simulink model "quaternion_pid_development_sim"  (R2025b)
settings: Solver=FixedStepAuto  StartTime=0.0  StopTime=tspan  FixedStep=dt_sim  RelTol=1e-3
values from neighbouring files (symbols this model uses):
  dt_data = round((dt_data_target/dt_sim))*dt_sim    [quaternion_pid_development.m]
  Kd = 0    [quaternion_pid_development.m]
  Ki = 0    [quaternion_pid_development.m]
  Kp = 3    [quaternion_pid_development.m]
  qib_0 = eulToQuat(Eul_0)    [quaternion_pid_development.m]
  qib_u = squeeze(results.qib_u.Data)'    [quaternion_pid_development.m]
settings Model: Creator=koryh  LastModifiedBy=koryh

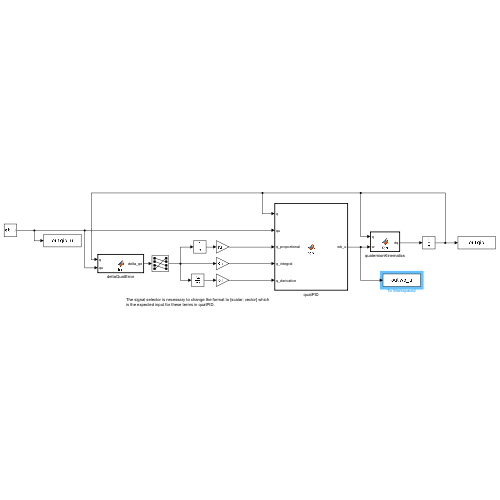
[thumbnail: Simulink's stored preview of the top-level diagram]
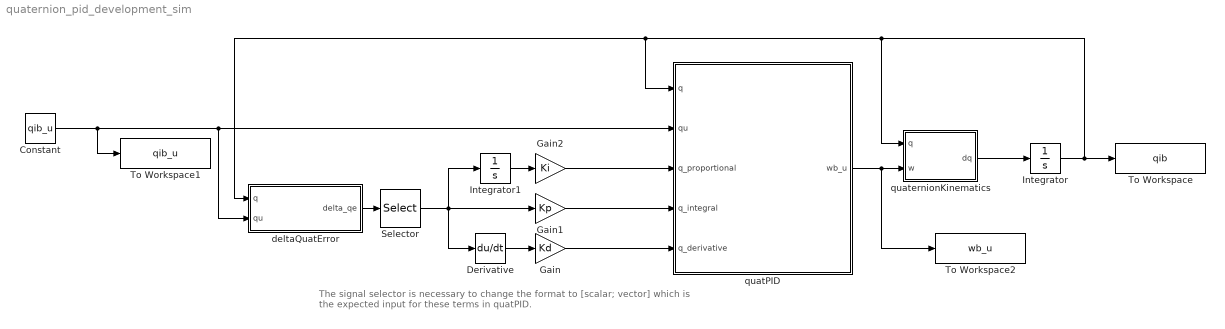
== system quaternion_pid_development_sim ==
  note: The signal selector is necessary to change the format to [scalar; vector] which
      | is the expected input for these terms in quatPID.
  Constant : Constant  Value=qib_u
  Derivative : Derivative
  Gain : Gain  Gain=Kd
  Gain1 : Gain  Gain=Kp
  Gain2 : Gain  Gain=Ki
  Integrator : Integrator  InitialCondition=qib_0
  Integrator1 : Integrator
  Selector : Selector  InputPortWidth=4  IndexOptions=Index vector (dialog)  Indices=[4 1 2 3]  OutputSizes=1
  To Workspace : ToWorkspace  VariableName=qib  SaveFormat=Timeseries  SampleTime=dt_data
  To Workspace1 : ToWorkspace  VariableName=qib_u  SaveFormat=Timeseries  SampleTime=dt_data
  To Workspace2 : ToWorkspace  VariableName=wb_u  SaveFormat=Timeseries  SampleTime=dt_data
  deltaQuatError : MATLAB Function  TreatAsAtomicUnit=on
  quatPID : MATLAB Function  TreatAsAtomicUnit=on
  quaternionKinematics : MATLAB Function  TreatAsAtomicUnit=on
  wires:
  quaternionKinematics/1(dq) -> Integrator/1
  quatPID/1(wb_u) -> quaternionKinematics/2(w), To Workspace2/1
  Constant/1 -> deltaQuatError/2(qu), quatPID/2(qu), To Workspace1/1
  deltaQuatError/1(delta_qe) -> Selector/1
  Selector/1 -> Integrator1/1, Gain1/1, Derivative/1
  Derivative/1 -> Gain/1
  Gain/1 -> quatPID/5(q_derivative)
  Integrator1/1 -> Gain2/1
  Gain2/1 -> quatPID/3(q_proportional)
  Gain1/1 -> quatPID/4(q_integral)
  Integrator/1 -> To Workspace/1, quaternionKinematics/1(q), quatPID/1(q), deltaQuatError/1(q)

== matlab function quaternion_pid_development_sim/deltaQuatError ==
  data: q input; delta_qe output; qu input
function delta_qe = fcn(q, qu)

delta_qe = deltaQuatError(q, qu);

== matlab function quaternion_pid_development_sim/quatPID ==
  data: q input; wb_u output; qu input; q_proportional input; q_integral input; q_derivative input
function wb_u = fcn(q, qu, q_proportional, q_integral, q_derivative)

wb_u = quatPID(q, qu, q_proportional, q_integral, q_derivative);

== matlab function quaternion_pid_development_sim/quaternionKinematics ==
  data: q input; dq output; w input
function dq = fcn(q,w)

%Expects q as [vector; scalar]
dq = quaternionKinematics(q,w);
